simulink model "lego_selfbalance_custom"  (Simulink 8.2)
settings: Solver=ode3  SolverMode=SingleTasking  StartTime=0.0  StopTime=inf  FixedStep=0.004  MaxStep=TS  RelTol=1e-3
PostLoadFcn:
  | lego_selfbalance_plant;
  | lego_selfbalance_controller;
  | lego_selfbalance_simulation;
InitFcn:
  | lego_selfbalance_plant;
  | lego_selfbalance_controller;
  | lego_selfbalance_simulation;
  | 
  | lego_drive_selfbalance_InitData.mdl = get_param(bdroot,'Name');
  | lego_drive_selfbalance_InitData.cs = getActiveConfigSet(lego_drive_selfbalance_InitData.mdl);
values from neighbouring files (symbols this model uses):
  A1 = [ ... (first row only)    [lego_selfbalance_plant.m]
  A2 = [ ... (first row only)    [lego_selfbalance_plant.m]
  B1 = [ ... (first row only)    [lego_selfbalance_plant.m]
  B2 = [ ... (first row only)    [lego_selfbalance_plant.m]
  BATTERY = 8000    [lego_selfbalance_simulation.m]
  C1 = eye(4)    [lego_selfbalance_plant.m]
  C2 = eye(2)    [lego_selfbalance_plant.m]
  D = 0.04    [lego_selfbalance_plant.m]
  D1 = zeros(4, 2)    [lego_selfbalance_plant.m]
  D2 = zeros(2)    [lego_selfbalance_plant.m]
  GYRO0 = 600    [lego_selfbalance_simulation.m]
  R = 0.04    [lego_selfbalance_plant.m]
  START_POS = [100, 100]    [lego_selfbalance_simulation.m]
  TS = 0.001    [lego_selfbalance_simulation.m]
  W = 0.14    [lego_selfbalance_plant.m]
  X1IV = [ ... (first row only)    [lego_selfbalance_simulation.m]
  X2IV = [ ... (first row only)    [lego_selfbalance_simulation.m]
undefined symbols (not defined in the file or in its folder): a_b, a_d, a_gc, a_gd, a_r, DiscIntNeverNeededParam, k_f, k_i, k_sync, pwm_gain, pwm_offset, time_start, ts1, Turn
libraries: legonxtlib x11, simulink x4, realtime_examples_misc x1
PreSaveFcn:
  | set_param(gcs, 'Location',[35 56 895 605])
CloseFcn:
  | clear lego_drive_selfbalance_InitData
  | lego_selfbalance_closemodel
settings Model: Creator=The MathWorks Inc.  LastModifiedBy=Alphonso Monk  ExtModeTrigDuration=2
settings OptimizationCC: OptimizeModelRefInitCode=on  LifeSpan=1
settings DebuggingCC: SolverPrmCheckMsg=none  SingleTaskRateTransMsg=warning  Int32ToFloatConvMsg=none  ParameterPrecisionLossMsg=none
settings HardwareCC: ProdLargestAtomicInteger=Long  ProdLargestAtomicFloat=Float  ProdEndianess=LittleEndian  ProdHWDeviceType=ARM Compatible->ARM 7
settings SFSimCC: SimParseCustomCode=off
settings RTWCC: SystemTargetFile=realtime.tlc  GenCodeOnly=on  GenerateMakefile=off  TemplateMakefile=realtime.tmf  Description=Run on Target Hardware  RTWVerbose=off  ProcessScript=realtime_make_rtw_hook
settings CodeAppCC: CustomSymbolStrType=$N$R$M  InternalIdentifier=Classic
settings STFCustomTargetCC: TargetLibSuffix=.a  CodeReplacementLibrary=ANSI_C  GenerateSampleERTMain=on  ERTCustomFileBanners=on  SupportNonInlinedSFcns=off  SupportVariableSizeSignals=on  MATLABClassNameForMDSCustomization=Simulink.SoftwareTarget.ERTCustomization  GRTInterface=off  SystemTargetFile=realtime.tlc
settings ERTTargetCC: CodeReplacementLibrary=ANSI_C  MultiwordLength=2048  GenerateSampleERTMain=on  ParMdlRefBuildCompliant=off  CompOptLevelCompliant=off  ConcurrentExecutionCompliant=off  CombineOutputUpdateFcns=off  ERTFirstTimeCompliant=off  SupportContinuousTime=on  SupportVariableSizeSignals=on  ModelStepFunctionPrototypeControlCompliant=off  CPPClassGenCompliant=off  ExtModeTransport=1  ExtModeMexFile=ext_serial_win32_comm_no_acks_rtt_byteswap  ExtModeMexArgs=0 16 9600  InlinedParameterPlacement=NonHierarchical  ERTSrcFileBannerTemplate=realtime_code_template.cgt  ERTHdrFileBannerTemplate=realtime_code_template.cgt  ERTDataSrcFileTemplate=realtime_code_template.cgt  ERTDataHdrFileTemplate=realtime_code_template.cgt  ERTCustomFileTemplate=realtime_file_process.tlc  ConvertIfToSwitch=off  SuppressUnreachableDefaultCases=off
settings SettingsController: Description=Run on Hardware Dialog  TargetExtensionPlatform=LEGO MINDSTORMS NXT
settings MATStruct: Find_com_port=[0.0]  Enable_overrun_detection=[0.0]  Enable_LEGO_to_LEGO_communication=[1.0]  Bluetooth_mode=[1.0]  Slave_bluetooth_address=00:16:53:0f:0c:09

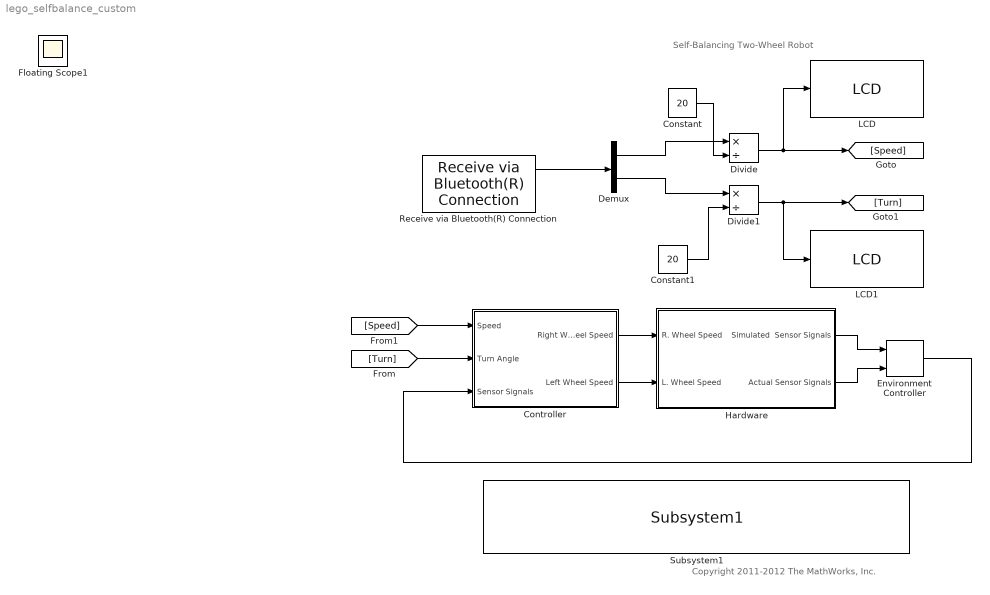
== system lego_selfbalance_custom ==
  note: Copyright 2011-2012 The MathWorks, Inc.
  note: Self-Balancing Two-Wheel Robot
  Constant : Constant  Value=20
  Constant1 : Constant  Value=20
  Controller : Subsystem  TreatAsAtomicUnit=on
  Demux : Demux  Outputs=2
  Divide : Product  Inputs=*/  OutDataTypeStr=single
  Divide1 : Product  Inputs=*/  OutDataTypeStr=single
  Environment Controller : simulink/Signal Routing/Environment Controller
  Hardware : Subsystem  VariantControl=DoSim
  LCD : legonxtlib/LCD  slcdStr=Speed  slcdLine=1  slcdFormat=Decimal
  LCD1 : legonxtlib/LCD  slcdStr=Turn:  slcdLine=2  slcdFormat=Decimal
  Receive via Bluetooth(R) Connection : legonxtlib/Receive via Bluetooth(R) Connection  mailbox=1  dataType=int32  dataSize=2  sampleTime=0.048
  Subsystem1 : realtime_examples_misc/Subsystem1  SystemSampleTime=-1
  Floating Scope1 : Scope
      settings: Floating=on  YMin=0  YMax=70000
  wires:
  Environment Controller/1 -> Controller/3(Sensor Signals)
  Controller/1(Right Wheel Speed) -> Hardware/1(R. Wheel Speed)
  Controller/2(Left Wheel Speed) -> Hardware/2(L. Wheel Speed)
  Hardware/1(Simulated  Sensor Signals) -> Environment Controller/1
  Hardware/2(Actual Sensor Signals) -> Environment Controller/2
  Constant/1 -> Divide/2
  Receive via Bluetooth(R) Connection/1 -> Demux/1
  Demux/1 -> Divide/1
  Constant1/1 -> Divide1/2
  Demux/2 -> Divide1/1
  Divide/1 -> [Speed], LCD/1
  Divide1/1 -> [Turn], LCD1/1
  [Turn] -> Controller/2(Turn Angle)
  [Speed] -> Controller/1(Speed)

== system lego_selfbalance_custom/Controller ==
  Speed : Inport
  Turn Angle : Inport  Port=2
  Sensor Signals : Inport  Port=3
  Balance and Drive Control : Subsystem
  Compare To Constant : simulink/Logic and Bit Operations/Compare To Constant  relop=>=  const=time_start  OutDataTypeStr=boolean
  Demux : Demux  Outputs=5
  Gyro Calibration : Subsystem  TreatAsAtomicUnit=on
  Logical Operator : Logic  Operator=NOT  AllPortsSameDT=off  OutDataTypeStr=boolean
  Right Wheel Speed : Outport
  Left Wheel Speed : Outport  Port=2
  wires:
  Compare To Constant/1 -> Logical Operator/1, Balance and Drive Control/Enable
  Gyro Calibration/1(Gyro Offset) -> Balance and Drive Control/1(Gyro Offset)
  Logical Operator/1 -> Gyro Calibration/Enable
  Sensor Signals/1 -> Demux/1
  Demux/4 -> Gyro Calibration/1(Gyro), Balance and Drive Control/2(Gyro)
  Speed/1 -> Balance and Drive Control/3(Speed)
  Turn Angle/1 -> Balance and Drive Control/4(Turn Angle)
  Demux/5 -> Balance and Drive Control/7(Battery)
  Demux/3 -> Balance and Drive Control/6(L. Wheel Rotation)
  Demux/2 -> Balance and Drive Control/5(R. Wheel Rotation)
  Demux/1 -> Compare To Constant/1
  Balance and Drive Control/1(R. Wheel Speed) -> Right Wheel Speed/1
  Balance and Drive Control/2(L. Wheel Speed) -> Left Wheel Speed/1

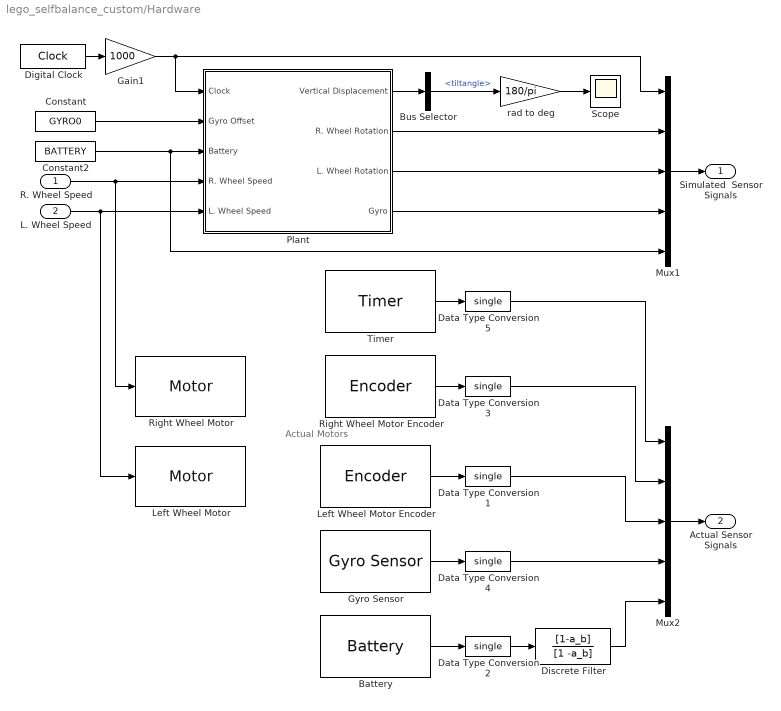
== system lego_selfbalance_custom/Hardware ==
  note: Actual
      | Motors
  R. Wheel Speed : Inport
  L. Wheel Speed : Inport  Port=2
  Battery : legonxtlib/Battery  sampleTime=ts1
  Bus Selector : BusSelector  OutputSignals=tiltangle
  Constant : Constant  Value=GYRO0  OutDataTypeStr=single
  Constant2 : Constant  Value=BATTERY  OutDataTypeStr=single
  Data Type Conversion{1..5} (5 alike) : DataTypeConversion  OutDataTypeStr=single  RndMeth=Simplest
  Digital Clock : DigitalClock  SampleTime=4*TS
  Discrete Filter : DiscreteFilter  Numerator=[1-a_b]  Denominator=[1 -a_b]
  Gain1 : Gain  Gain=1000  OutDataTypeStr=single  ParamDataTypeStr=Inherit: Same as input
  Gyro Sensor : legonxtlib/Gyro Sensor  portNumber=4  outputMode=Raw A/D (0 - 1023)  offset=600  sampleTime=ts1
  Left Wheel Motor : legonxtlib/Motor  sportNumber=C  sstopAction=Brake
  Left Wheel Motor Encoder : legonxtlib/Encoder  portNumber=C  opMode=No reset  sampleTime=ts1
  Mux1 : Mux  Inputs=5
  Mux2 : Mux  Inputs=5
  Plant : Subsystem
  Right Wheel Motor : legonxtlib/Motor  sportNumber=B  sstopAction=Brake
  Right Wheel Motor Encoder : legonxtlib/Encoder  portNumber=B  opMode=No reset  sampleTime=ts1
  Scope : Scope
      settings: YMin=-90  YMax=90
  Timer : legonxtlib/Timer  sampleTime=ts1
  rad to deg : Gain  Gain=180/pi
  Simulated  Sensor Signals : Outport
  Actual Sensor Signals : Outport  Port=2
  wires:
  Data Type Conversion5/1 -> Mux2/1
  Timer/1 -> Data Type Conversion5/1
  Data Type Conversion4/1 -> Mux2/4
  Data Type Conversion1/1 -> Mux2/3
  Data Type Conversion3/1 -> Mux2/2
  Mux2/1 -> Actual Sensor Signals/1
  Left Wheel Motor Encoder/1 -> Data Type Conversion1/1
  Right Wheel Motor Encoder/1 -> Data Type Conversion3/1
  Battery/1 -> Data Type Conversion2/1
  Data Type Conversion2/1 -> Discrete Filter/1
  Discrete Filter/1 -> Mux2/5
  Gyro Sensor/1 -> Data Type Conversion4/1
  L. Wheel Speed/1 -> Plant/5(L. Wheel Speed), Left Wheel Motor/1
  Mux1/1 -> Simulated  Sensor Signals/1
  Plant/3(L. Wheel Rotation) -> Mux1/3
  R. Wheel Speed/1 -> Plant/4(R. Wheel Speed), Right Wheel Motor/1
  Constant2/1 -> Mux1/5, Plant/3(Battery)
  Plant/2(R. Wheel Rotation) -> Mux1/2
  Plant/4(Gyro) -> Mux1/4
  Digital Clock/1 -> Gain1/1
  Gain1/1 -> Mux1/1, Plant/1(Clock)
  rad to deg/1 -> Scope/1
  Plant/1(Vertical Displacement) -> Bus Selector/1
  Bus Selector/1 -> rad to deg/1  "<tiltangle>"
  Constant/1 -> Plant/2(Gyro Offset)

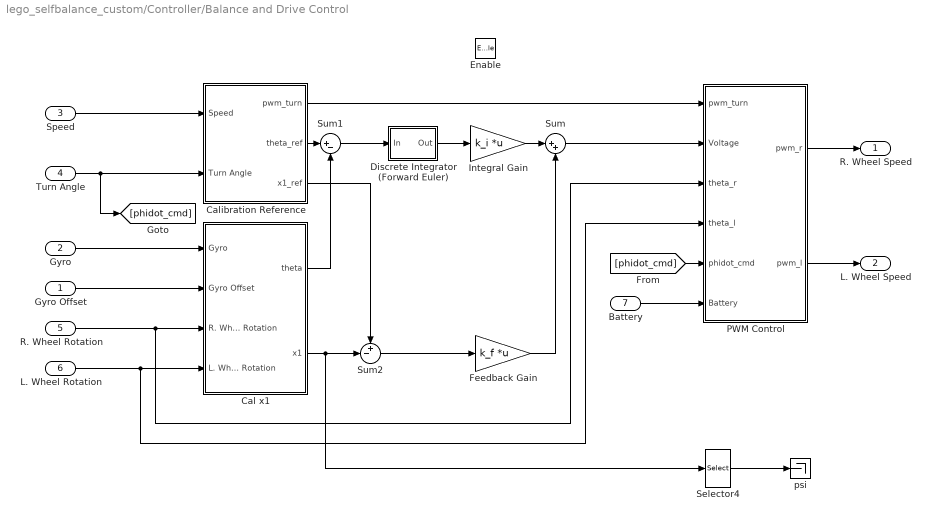
== system lego_selfbalance_custom/Controller/Balance and Drive Control ==
  Gyro Offset : Inport
  Gyro : Inport  Port=2
  Speed : Inport  Port=3
  Turn Angle : Inport  Port=4
  R. Wheel Rotation : Inport  Port=5
  L. Wheel Rotation : Inport  Port=6
  Battery : Inport  Port=7
  Enable : EnablePort
  Cal x1 : Subsystem
  Calibration Reference : Subsystem
  Discrete Integrator (Forward Euler) : Subsystem
  Feedback Gain : Gain  Gain=k_f  Multiplication=Matrix(K*u)  OutDataTypeStr=Inherit: Same as input  ParamDataTypeStr=Inherit: Same as input
  Integral Gain : Gain  Gain=k_i  Multiplication=Matrix(K*u)  OutDataTypeStr=Inherit: Same as input  ParamDataTypeStr=Inherit: Same as input
  PWM Control : Subsystem
  Selector4 : Selector  InputPortWidth=4  IndexOptions=Index vector (dialog)  Indices=2  OutputSizes=1
  Sum : Sum  Inputs=|++  OutDataTypeStr=Inherit: Same as first input
  Sum1 : Sum  Inputs=|+-  OutDataTypeStr=Inherit: Same as first input
  Sum2 : Sum  Inputs=+-|  OutDataTypeStr=Inherit: Same as first input
  psi : Terminator
  R. Wheel Speed : Outport
  L. Wheel Speed : Outport  Port=2
  wires:
  [phidot_cmd] -> PWM Control/5(phidot_cmd)
  Selector4/1 -> psi/1
  Calibration Reference/3(x1_ref) -> Sum2/1
  Sum2/1 -> Feedback Gain/1
  Cal x1/2(x1) -> Selector4/1, Sum2/2
  Integral Gain/1 -> Sum/1
  Discrete Integrator (Forward Euler)/1(Out) -> Integral Gain/1
  Sum1/1 -> Discrete Integrator (Forward Euler)/1(In)
  Cal x1/1(theta) -> Sum1/2
  Calibration Reference/2(theta_ref) -> Sum1/1
  Feedback Gain/1 -> Sum/2
  L. Wheel Rotation/1 -> PWM Control/4(theta_l), Cal x1/4(L. Wheel Rotation)
  Battery/1 -> PWM Control/6(Battery)
  Sum/1 -> PWM Control/2(Voltage)
  Turn Angle/1 -> [phidot_cmd], Calibration Reference/2(Turn Angle)
  Speed/1 -> Calibration Reference/1(Speed)
  Calibration Reference/1(pwm_turn) -> PWM Control/1(pwm_turn)
  PWM Control/1(pwm_r) -> R. Wheel Speed/1
  PWM Control/2(pwm_l) -> L. Wheel Speed/1
  R. Wheel Rotation/1 -> PWM Control/3(theta_r), Cal x1/3(R. Wheel Rotation)
  Gyro/1 -> Cal x1/1(Gyro)
  Gyro Offset/1 -> Cal x1/2(Gyro Offset)

== system lego_selfbalance_custom/Controller/Gyro Calibration ==
  note: Calculate gyro offset
  Gyro : Inport
  Enable : EnablePort
  Constant : Constant  Value=440  OutDataTypeStr=uint32  SampleTime=0.2
  Gain2 : Gain  Gain=1-a_gc  OutDataTypeStr=Inherit: Same as input  ParamDataTypeStr=Inherit: Same as input
  Gain3 : Gain  Gain=a_gc  OutDataTypeStr=Inherit: Same as input  ParamDataTypeStr=Inherit: Same as input
  Speaker : legonxtlib/Speaker  sinputMode=Frequency only  sspeakerFreq=100  sspeakerVolume=80  sspeakerDuration=100
  Sum1 : Sum  Inputs=|++  OutDataTypeStr=Inherit: Same as first input
  Unit Delay : UnitDelay  SampleTime=-1
  Gyro Offset : Outport
  wires:
  Gain3/1 -> Sum1/2
  Unit Delay/1 -> Gain3/1
  Sum1/1 -> Unit Delay/1, Gyro Offset/1
  Gain2/1 -> Sum1/1
  Gyro/1 -> Gain2/1
  Constant/1 -> Speaker/1

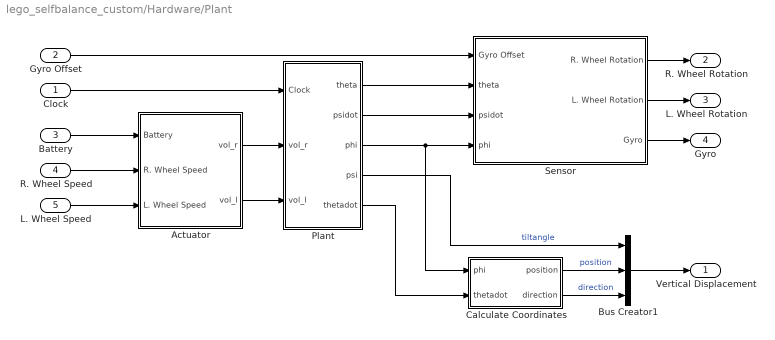
== system lego_selfbalance_custom/Hardware/Plant ==
  Clock : Inport
  Gyro Offset : Inport  Port=2
  Battery : Inport  Port=3
  R. Wheel Speed : Inport  Port=4
  L. Wheel Speed : Inport  Port=5
  Actuator : Subsystem
  Bus Creator1 : BusCreator  Inputs=3
  Calculate Coordinates : Subsystem
  Plant : Subsystem
  Sensor : Subsystem
  Vertical Displacement : Outport
  R. Wheel Rotation : Outport  Port=2
  L. Wheel Rotation : Outport  Port=3
  Gyro : Outport  Port=4
  wires:
  Clock/1 -> Plant/1(Clock)
  Plant/4(psi) -> Bus Creator1/1  "tiltangle"
  Bus Creator1/1 -> Vertical Displacement/1
  Calculate Coordinates/2(direction) -> Bus Creator1/3  "direction"
  Calculate Coordinates/1(position) -> Bus Creator1/2  "position"
  Plant/3(phi) -> Calculate Coordinates/1(phi), Sensor/4(phi)
  L. Wheel Speed/1 -> Actuator/3(L. Wheel Speed)
  Plant/5(thetadot) -> Calculate Coordinates/2(thetadot)
  Sensor/3(Gyro) -> Gyro/1
  R. Wheel Speed/1 -> Actuator/2(R. Wheel Speed)
  Sensor/2(L. Wheel Rotation) -> L. Wheel Rotation/1
  Sensor/1(R. Wheel Rotation) -> R. Wheel Rotation/1
  Gyro Offset/1 -> Sensor/1(Gyro Offset)
  Battery/1 -> Actuator/1(Battery)
  Plant/1(theta) -> Sensor/2(theta)
  Plant/2(psidot) -> Sensor/3(psidot)
  Actuator/2(vol_l) -> Plant/3(vol_l)
  Actuator/1(vol_r) -> Plant/2(vol_r)

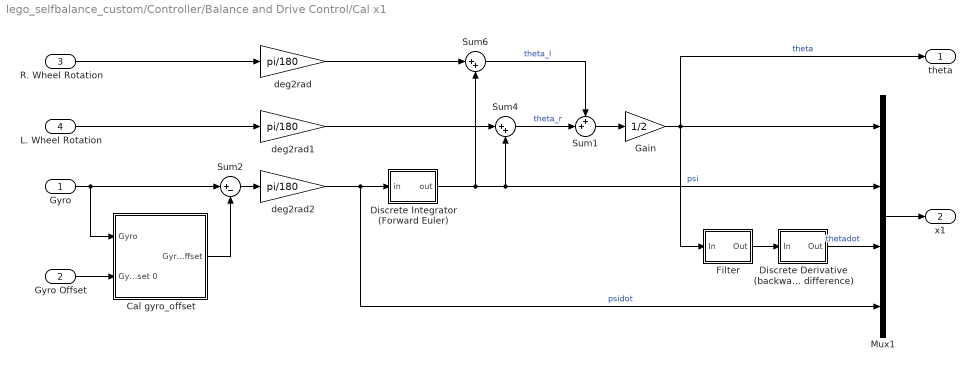
== system lego_selfbalance_custom/Controller/Balance and Drive Control/Cal x1 ==
  Gyro : Inport
  Gyro Offset : Inport  Port=2
  R. Wheel Rotation : Inport  Port=3
  L. Wheel Rotation : Inport  Port=4
  Cal gyro_offset : Subsystem
  Discrete Derivative (backward difference) : Subsystem
  Discrete Integrator (Forward Euler) : Subsystem
  Filter : Subsystem
  Gain : Gain  Gain=1/2  OutDataTypeStr=Inherit: Same as input  ParamDataTypeStr=Inherit: Same as input
  Mux1 : Mux
  Sum1 : Sum  Inputs=++|  OutDataTypeStr=Inherit: Same as first input
  Sum2 : Sum  Inputs=|+-  OutDataTypeStr=Inherit: Same as first input
  Sum4 : Sum  Inputs=|++  OutDataTypeStr=Inherit: Same as first input
  Sum6 : Sum  Inputs=|++  OutDataTypeStr=Inherit: Same as first input
  deg2rad : Gain  Gain=pi/180  OutDataTypeStr=Inherit: Same as input  ParamDataTypeStr=Inherit: Same as input
  deg2rad1 : Gain  Gain=pi/180  OutDataTypeStr=Inherit: Same as input  ParamDataTypeStr=Inherit: Same as input
  deg2rad2 : Gain  Gain=pi/180  OutDataTypeStr=Inherit: Same as input  ParamDataTypeStr=Inherit: Same as input
  theta : Outport
  x1 : Outport  Port=2
  wires:
  Gain/1 -> Mux1/1, theta/1, Filter/1(In)  "theta"
  Filter/1(Out) -> Discrete Derivative (backward difference)/1(In)
  deg2rad2/1 -> Mux1/4, Discrete Integrator (Forward Euler)/1(in)  "psidot"
  Sum1/1 -> Gain/1
  Sum4/1 -> Sum1/2  "theta_r"
  Sum6/1 -> Sum1/1  "theta_l"
  Discrete Derivative (backward difference)/1(Out) -> Mux1/3  "thetadot"
  L. Wheel Rotation/1 -> deg2rad1/1
  R. Wheel Rotation/1 -> deg2rad/1
  deg2rad/1 -> Sum6/1
  Discrete Integrator (Forward Euler)/1(out) -> Mux1/2, Sum4/2, Sum6/2  "psi"
  Mux1/1 -> x1/1
  deg2rad1/1 -> Sum4/1
  Gyro/1 -> Sum2/1, Cal gyro_offset/1(Gyro)
  Sum2/1 -> deg2rad2/1
  Cal gyro_offset/1(Gyro Offset) -> Sum2/2
  Gyro Offset/1 -> Cal gyro_offset/2(Gyro Offset 0)

== system lego_selfbalance_custom/Controller/Balance and Drive Control/Calibration Reference ==
  note: thetadot_cmd should be
      | between 0 and 7.5
  note: phidot_cmd should be
      | between 0 and 25
  Speed : Inport
  Turn Angle : Inport  Port=2
  Constant2 : Constant  Value=0  VectorParams1D=off  OutDataTypeStr=single
  Constant3 : Constant  Value=0  VectorParams1D=off  OutDataTypeStr=single
  Discrete Integrator (Forward Euler) : Subsystem
  Filter : Subsystem
  Mux : Mux
  pwm_turn : Outport
  theta_ref : Outport  Port=2
  x1_ref : Outport  Port=3
  wires:
  Filter/1(out) -> Mux/3, Discrete Integrator (Forward Euler)/1(in)  "thetadot_ref"
  Constant3/1 -> Mux/4  "psidot_ref"
  Constant2/1 -> Mux/2  "psi_ref"
  Discrete Integrator (Forward Euler)/1(out) -> Mux/1, theta_ref/1  "theta_ref"
  Mux/1 -> x1_ref/1
  Turn Angle/1 -> pwm_turn/1
  Speed/1 -> Filter/1(in)

== system lego_selfbalance_custom/Controller/Balance and Drive Control/Discrete Integrator (Forward Euler) ==
  In : Inport
  Gain : Gain  Gain=ts1  OutDataTypeStr=Inherit: Same as input  ParamDataTypeStr=Inherit: Same as input
  Sum : Sum  Inputs=|++  OutDataTypeStr=Inherit: Same as first input
  Unit Delay : UnitDelay  SampleTime=-1
  Out : Outport
  wires:
  In/1 -> Gain/1
  Sum/1 -> Unit Delay/1
  Gain/1 -> Sum/1
  Unit Delay/1 -> Out/1, Sum/2

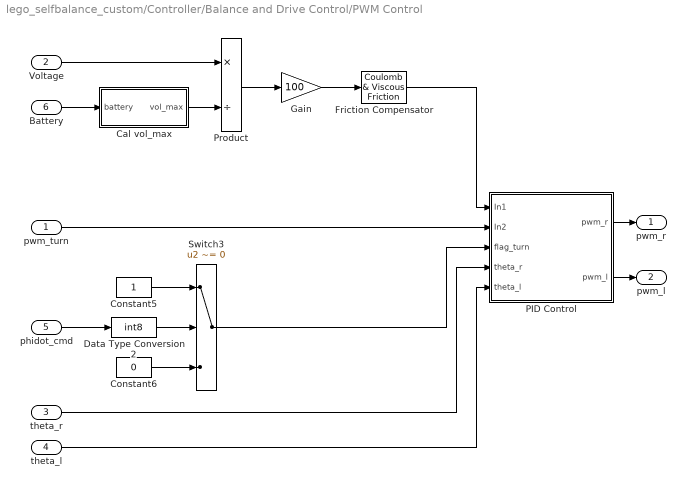
== system lego_selfbalance_custom/Controller/Balance and Drive Control/PWM Control ==
  pwm_turn : Inport
  Voltage : Inport  Port=2
  theta_r : Inport  Port=3
  theta_l : Inport  Port=4
  phidot_cmd : Inport  Port=5
  Battery : Inport  Port=6
  Cal vol_max : Subsystem
  Constant5 : Constant  OutDataTypeStr=boolean
  Constant6 : Constant  Value=0  OutDataTypeStr=boolean
  Data Type Conversion2 : DataTypeConversion  OutDataTypeStr=int8  RndMeth=Simplest
  Friction Compensator : simulink/Discontinuities/Coulomb & Viscous Friction  offset=pwm_offset  gain=pwm_gain
      settings: AttributesFormatString=gain = %<gain>\noffset = %<offset>
  Gain : Gain  Gain=100  OutDataTypeStr=Inherit: Same as input  ParamDataTypeStr=Inherit: Same as input
  PID Control : Subsystem
  Product : Product  Inputs=*/  RndMeth=Simplest  OutDataTypeStr=Inherit: Same as first input
  Switch3 : Switch  Criteria=u2 ~= 0
  pwm_r : Outport
  pwm_l : Outport  Port=2
  wires:
  Data Type Conversion2/1 -> Switch3/2
  phidot_cmd/1 -> Data Type Conversion2/1
  Constant6/1 -> Switch3/3
  Constant5/1 -> Switch3/1
  theta_l/1 -> PID Control/5(theta_l)
  theta_r/1 -> PID Control/4(theta_r)
  Cal vol_max/1(vol_max) -> Product/2
  Battery/1 -> Cal vol_max/1(battery)
  Product/1 -> Gain/1
  Voltage/1 -> Product/1
  Gain/1 -> Friction Compensator/1
  PID Control/1(pwm_r) -> pwm_r/1
  Friction Compensator/1 -> PID Control/1(In1)
  PID Control/2(pwm_l) -> pwm_l/1
  pwm_turn/1 -> PID Control/2(In2)
  Switch3/1 -> PID Control/3(flag_turn)

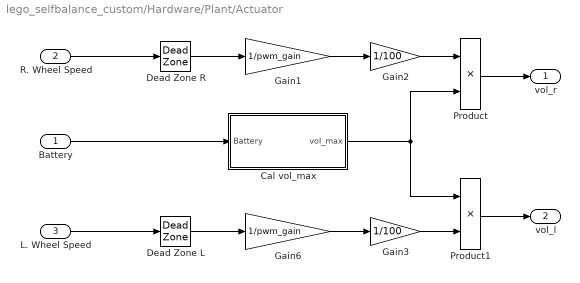
== system lego_selfbalance_custom/Hardware/Plant/Actuator ==
  Battery : Inport
  R. Wheel Speed : Inport  Port=2
  L. Wheel Speed : Inport  Port=3
  Cal vol_max : Subsystem
  Dead Zone L : DeadZone  LowerValue=-pwm_offset  UpperValue=pwm_offset  SaturateOnIntegerOverflow=on
      settings: AttributesFormatString=start=%<LowerValue>\nend=%<UpperValue>
  Dead Zone R : DeadZone  LowerValue=-pwm_offset  UpperValue=pwm_offset  SaturateOnIntegerOverflow=on
      settings: AttributesFormatString=start=%<LowerValue>\nend=%<UpperValue>
  Gain1 : Gain  Gain=1/pwm_gain  OutDataTypeStr=Inherit: Same as input  ParamDataTypeStr=Inherit: Same as input
  Gain2 : Gain  Gain=1/100  OutDataTypeStr=Inherit: Same as input  ParamDataTypeStr=Inherit: Same as input
  Gain3 : Gain  Gain=1/100  OutDataTypeStr=Inherit: Same as input  ParamDataTypeStr=Inherit: Same as input
  Gain6 : Gain  Gain=1/pwm_gain  OutDataTypeStr=Inherit: Same as input  ParamDataTypeStr=Inherit: Same as input
  Product : Product  RndMeth=Simplest
  Product1 : Product  RndMeth=Simplest
  vol_r : Outport
  vol_l : Outport  Port=2
  wires:
  Battery/1 -> Cal vol_max/1(Battery)
  Cal vol_max/1(vol_max) -> Product1/1, Product/2
  Dead Zone R/1 -> Gain1/1
  Product1/1 -> vol_l/1
  Gain3/1 -> Product1/2
  Product/1 -> vol_r/1
  Gain2/1 -> Product/1
  Gain6/1 -> Gain3/1
  Gain1/1 -> Gain2/1
  L. Wheel Speed/1 -> Dead Zone L/1
  R. Wheel Speed/1 -> Dead Zone R/1
  Dead Zone L/1 -> Gain6/1

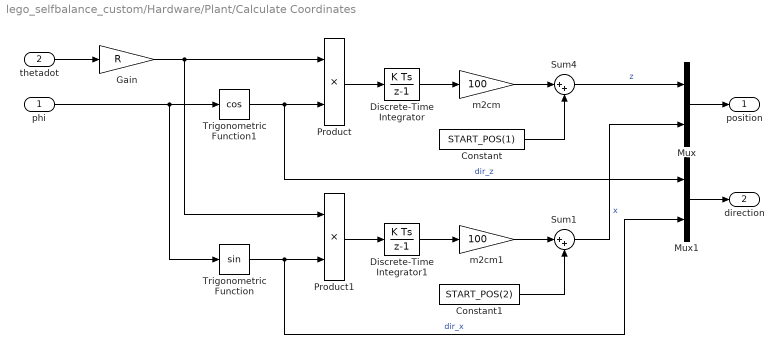
== system lego_selfbalance_custom/Hardware/Plant/Calculate Coordinates ==
  phi : Inport
  thetadot : Inport  Port=2
  Constant : Constant  Value=START_POS(1)  OutDataTypeStr=double
      settings: AttributesFormatString=DataType = %<OutDataTypeStr>
  Constant1 : Constant  Value=START_POS(2)  OutDataTypeStr=double
      settings: AttributesFormatString=DataType = %<OutDataTypeStr>
  Discrete-Time Integrator : DiscreteIntegrator  SampleTime=4*TS  ICPrevOutput=DiscIntNeverNeededParam  ICPrevScaledInput=DiscIntNeverNeededParam
  Discrete-Time Integrator1 : DiscreteIntegrator  SampleTime=4*TS  ICPrevOutput=DiscIntNeverNeededParam  ICPrevScaledInput=DiscIntNeverNeededParam
  Gain : Gain  Gain=R
  Mux : Mux  Inputs=2
  Mux1 : Mux  Inputs=2
  Product : Product  OutDataTypeStr=double  RndMeth=Simplest
  Product1 : Product  OutDataTypeStr=double  RndMeth=Simplest
  Sum1 : Sum  Inputs=|++
  Sum4 : Sum  Inputs=|++
  Trigonometric Function : Trigonometry
  Trigonometric Function1 : Trigonometry  Operator=cos
  m2cm : Gain  Gain=100
  m2cm1 : Gain  Gain=100
  position : Outport
  direction : Outport  Port=2
  wires:
  Mux1/1 -> direction/1
  Mux/1 -> position/1
  Sum1/1 -> Mux/2  "x"
  Constant1/1 -> Sum1/2
  m2cm1/1 -> Sum1/1
  Constant/1 -> Sum4/2
  Sum4/1 -> Mux/1  "z"
  m2cm/1 -> Sum4/1
  Gain/1 -> Product/1, Product1/1
  Discrete-Time Integrator1/1 -> m2cm1/1
  Discrete-Time Integrator/1 -> m2cm/1
  phi/1 -> Trigonometric Function/1, Trigonometric Function1/1
  thetadot/1 -> Gain/1
  Trigonometric Function1/1 -> Mux1/1, Product/2  "dir_z"
  Product/1 -> Discrete-Time Integrator/1
  Trigonometric Function/1 -> Mux1/2, Product1/2  "dir_x"
  Product1/1 -> Discrete-Time Integrator1/1

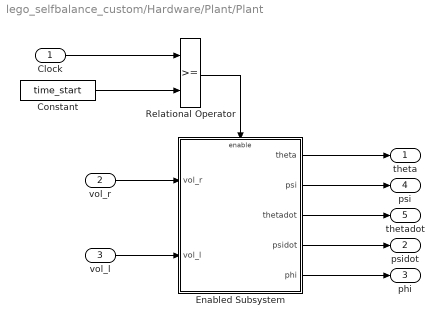
== system lego_selfbalance_custom/Hardware/Plant/Plant ==
  Clock : Inport
  vol_r : Inport  Port=2
  vol_l : Inport  Port=3
  Constant : Constant  Value=time_start  OutDataTypeStr=single
  Enabled Subsystem : Subsystem  TreatAsAtomicUnit=on
      settings: MinAlgLoopOccurrences=on
  Relational Operator : RelationalOperator  OutDataTypeStr=boolean
  theta : Outport
  psidot : Outport  Port=2
  phi : Outport  Port=3
  psi : Outport  Port=4
  thetadot : Outport  Port=5
  wires:
  Enabled Subsystem/4(psidot) -> psidot/1
  Enabled Subsystem/5(phi) -> phi/1
  Enabled Subsystem/2(psi) -> psi/1
  Enabled Subsystem/3(thetadot) -> thetadot/1
  Enabled Subsystem/1(theta) -> theta/1
  Constant/1 -> Relational Operator/2
  Clock/1 -> Relational Operator/1
  Relational Operator/1 -> Enabled Subsystem/Enable
  vol_l/1 -> Enabled Subsystem/2(vol_l)
  vol_r/1 -> Enabled Subsystem/1(vol_r)

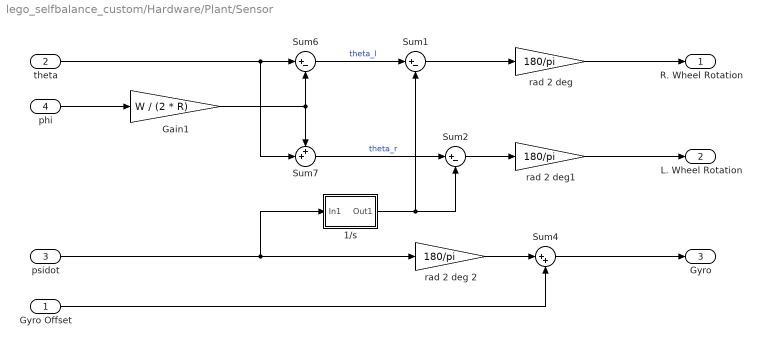
== system lego_selfbalance_custom/Hardware/Plant/Sensor ==
  Gyro Offset : Inport
  theta : Inport  Port=2
  psidot : Inport  Port=3
  phi : Inport  Port=4
  1/s : Subsystem
  Gain1 : Gain  Gain=W / (2 * R)
  Sum1 : Sum  Inputs=|+-
  Sum2 : Sum  Inputs=|+-
  Sum4 : Sum  Inputs=|++
  Sum6 : Sum  Inputs=|+-
  Sum7 : Sum  Inputs=++|
  rad 2 deg : Gain  Gain=180/pi  OutDataTypeStr=single
  rad 2 deg 2 : Gain  Gain=180/pi
  rad 2 deg1 : Gain  Gain=180/pi  OutDataTypeStr=single
  R. Wheel Rotation : Outport
  L. Wheel Rotation : Outport  Port=2
  Gyro : Outport  Port=3
  wires:
  1/s/1(Out1) -> Sum1/2, Sum2/2
  Sum6/1 -> Sum1/1  "theta_l"
  rad 2 deg1/1 -> L. Wheel Rotation/1
  rad 2 deg/1 -> R. Wheel Rotation/1
  Sum2/1 -> rad 2 deg1/1
  psidot/1 -> 1/s/1(In1), rad 2 deg 2/1
  Sum1/1 -> rad 2 deg/1
  Gain1/1 -> Sum6/2, Sum7/1
  phi/1 -> Gain1/1
  theta/1 -> Sum6/1, Sum7/2
  rad 2 deg 2/1 -> Sum4/1
  Sum7/1 -> Sum2/1  "theta_r"
  Gyro Offset/1 -> Sum4/2
  Sum4/1 -> Gyro/1

== system lego_selfbalance_custom/Controller/Balance and Drive Control/Cal x1/Cal gyro_offset ==
  Gyro : Inport
  Gyro Offset 0 : Inport  Port=2
  Gain1 : Gain  Gain=1-a_gd  OutDataTypeStr=Inherit: Same as input  ParamDataTypeStr=Inherit: Same as input
  Gain4 : Gain  Gain=a_gd  OutDataTypeStr=Inherit: Same as input  ParamDataTypeStr=Inherit: Same as input
  Sum2 : Sum  Inputs=|++  OutDataTypeStr=Inherit: Same as first input
  Unit Delay External IC : simulink/Additional Math & Discrete/Additional Discrete/Unit Delay External IC  tsamp=-1
  Gyro Offset : Outport
  wires:
  Gyro/1 -> Gain1/1
  Gyro Offset 0/1 -> Unit Delay External IC/2
  Gain1/1 -> Sum2/1
  Sum2/1 -> Gyro Offset/1, Unit Delay External IC/1
  Unit Delay External IC/1 -> Gain4/1
  Gain4/1 -> Sum2/2

== system lego_selfbalance_custom/Controller/Balance and Drive Control/Cal x1/Discrete Derivative (backward difference) ==
  In : Inport
  Gain : Gain  Gain=1/ts1  OutDataTypeStr=Inherit: Same as input  ParamDataTypeStr=Inherit: Same as input
  Sum : Sum  Inputs=|+-  OutDataTypeStr=Inherit: Same as first input
  Unit Delay : UnitDelay  SampleTime=-1
  Out : Outport
  wires:
  Gain/1 -> Out/1
  In/1 -> Sum/1, Unit Delay/1
  Unit Delay/1 -> Sum/2
  Sum/1 -> Gain/1

== system lego_selfbalance_custom/Controller/Balance and Drive Control/Cal x1/Discrete Integrator (Forward Euler) ==
  in : Inport
  Gain : Gain  Gain=ts1  OutDataTypeStr=Inherit: Same as input  ParamDataTypeStr=Inherit: Same as input
  Sum : Sum  Inputs=|++  OutDataTypeStr=Inherit: Same as first input
  Unit Delay : UnitDelay  SampleTime=-1
  out : Outport
  wires:
  Unit Delay/1 -> Sum/2, out/1
  Gain/1 -> Sum/1
  Sum/1 -> Unit Delay/1
  in/1 -> Gain/1

== system lego_selfbalance_custom/Controller/Balance and Drive Control/Cal x1/Filter ==
  In : Inport
  Gain2 : Gain  Gain=a_d  OutDataTypeStr=Inherit: Same as input  ParamDataTypeStr=Inherit: Same as input
  Gain3 : Gain  Gain=1-a_d  OutDataTypeStr=Inherit: Same as input  ParamDataTypeStr=Inherit: Same as input
  Sum : Sum  Inputs=|++  OutDataTypeStr=Inherit: Same as first input
  Unit Delay : UnitDelay  SampleTime=-1
  Out : Outport
  wires:
  In/1 -> Gain3/1
  Gain3/1 -> Sum/1
  Gain2/1 -> Sum/2
  Unit Delay/1 -> Gain2/1
  Sum/1 -> Out/1, Unit Delay/1

== system lego_selfbalance_custom/Controller/Balance and Drive Control/Calibration Reference/Discrete Integrator (Forward Euler) ==
  in : Inport
  Gain : Gain  Gain=ts1  OutDataTypeStr=Inherit: Same as input  ParamDataTypeStr=Inherit: Same as input
  Sum : Sum  Inputs=|++  OutDataTypeStr=Inherit: Same as first input
  Unit Delay : UnitDelay  SampleTime=-1
  out : Outport
  wires:
  in/1 -> Gain/1
  Sum/1 -> Unit Delay/1
  Gain/1 -> Sum/1
  Unit Delay/1 -> out/1, Sum/2

== system lego_selfbalance_custom/Controller/Balance and Drive Control/Calibration Reference/Filter ==
  note: Filter Function:
      |               1-a_r
      |          ----------------
      |          1-a_r*z^(-1)
  in : Inport
  Gain2 : Gain  Gain=a_r  OutDataTypeStr=Inherit: Same as input  ParamDataTypeStr=Inherit: Same as input
  Gain3 : Gain  Gain=1-a_r  OutDataTypeStr=Inherit: Same as input  ParamDataTypeStr=Inherit: Same as input
  Sum : Sum  Inputs=|++  OutDataTypeStr=Inherit: Same as first input
  Unit Delay : UnitDelay  SampleTime=-1
  out : Outport
  wires:
  in/1 -> Gain3/1
  Gain3/1 -> Sum/1
  Gain2/1 -> Sum/2
  Unit Delay/1 -> Gain2/1
  Sum/1 -> out/1, Unit Delay/1

== system lego_selfbalance_custom/Controller/Balance and Drive Control/PWM Control/Cal vol_max ==
  battery : Inport
  Constant : Constant  Value=0.625  OutDataTypeStr=single
      settings: AttributesFormatString=DataType = %<OutDataTypeStr>
  Gain3 : Gain  Gain=0.001089  OutDataTypeStr=Inherit: Same as input  ParamDataTypeStr=Inherit: Same as input
  Sum2 : Sum  Inputs=|+-  OutDataTypeStr=Inherit: Same as first input
  vol_max : Outport
  wires:
  Gain3/1 -> Sum2/1
  Sum2/1 -> vol_max/1
  Constant/1 -> Sum2/2
  battery/1 -> Gain3/1

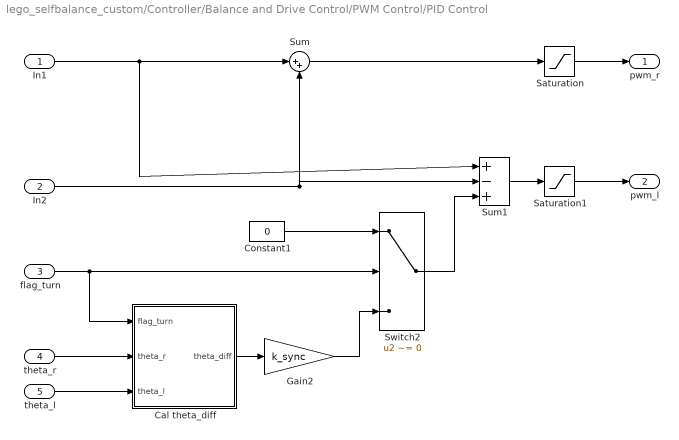
== system lego_selfbalance_custom/Controller/Balance and Drive Control/PWM Control/PID Control ==
  In1 : Inport
  In2 : Inport  Port=2
  flag_turn : Inport  Port=3
  theta_r : Inport  Port=4
  theta_l : Inport  Port=5
  Cal theta_diff : Subsystem
  Constant1 : Constant  Value=0  OutDataTypeStr=single
      settings: AttributesFormatString=DataType = %<OutDataTypeStr>
  Gain2 : Gain  Gain=k_sync  OutDataTypeStr=Inherit: Same as input  ParamDataTypeStr=Inherit: Same as input
  Saturation : Saturate  UpperLimit=100  LowerLimit=-100
      settings: AttributesFormatString=max = %<UpperLimit>\nmin = %<LowerLimit>
  Saturation1 : Saturate  UpperLimit=100  LowerLimit=-100
      settings: AttributesFormatString=max = %<UpperLimit>\nmin = %<LowerLimit>
  Sum : Sum  Inputs=|++  OutDataTypeStr=Inherit: Same as first input
  Sum1 : Sum  Inputs=|+-+  OutDataTypeStr=Inherit: Same as first input
  Switch2 : Switch  Criteria=u2 ~= 0
  pwm_r : Outport
  pwm_l : Outport  Port=2
  wires:
  In1/1 -> Sum1/1, Sum/1
  Gain2/1 -> Switch2/3
  Constant1/1 -> Switch2/1
  flag_turn/1 -> Switch2/2, Cal theta_diff/1(flag_turn)
  Cal theta_diff/1(theta_diff) -> Gain2/1
  Saturation/1 -> pwm_r/1
  Saturation1/1 -> pwm_l/1
  In2/1 -> Sum1/2, Sum/2
  Sum/1 -> Saturation/1
  theta_r/1 -> Cal theta_diff/2(theta_r)
  theta_l/1 -> Cal theta_diff/3(theta_l)
  Switch2/1 -> Sum1/3
  Sum1/1 -> Saturation1/1

== system lego_selfbalance_custom/Hardware/Plant/Actuator/Cal vol_max ==
  note: Calculate maximum DC motor (battery)
      | voltage using an experimental expression
  Battery : Inport
  Constant : Constant  Value=0.625  OutDataTypeStr=single
  Gain3 : Gain  Gain=0.001089  OutDataTypeStr=Inherit: Same as input  ParamDataTypeStr=Inherit: Same as input
  Sum2 : Sum  Inputs=|+-  OutDataTypeStr=Inherit: Same as first input
  vol_max : Outport
  wires:
  Constant/1 -> Sum2/2
  Sum2/1 -> vol_max/1
  Gain3/1 -> Sum2/1
  Battery/1 -> Gain3/1

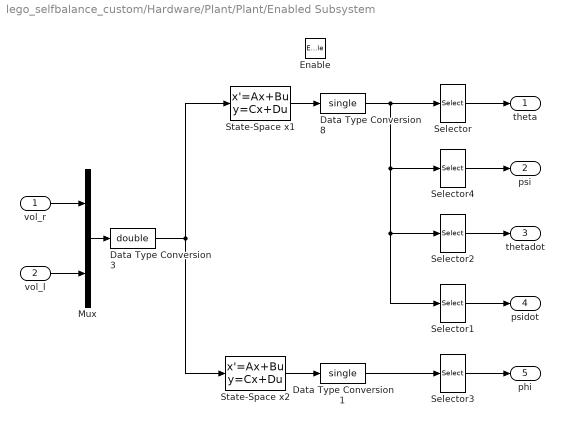
== system lego_selfbalance_custom/Hardware/Plant/Plant/Enabled Subsystem ==
  vol_r : Inport
  vol_l : Inport  Port=2
  Enable : EnablePort
  Data Type Conversion1 : DataTypeConversion  OutDataTypeStr=single  RndMeth=Nearest
  Data Type Conversion3 : DataTypeConversion  OutDataTypeStr=double  RndMeth=Nearest
  Data Type Conversion8 : DataTypeConversion  OutDataTypeStr=single  RndMeth=Nearest
  Mux : Mux  Inputs=2
  Selector : Selector  InputPortWidth=4  IndexOptions=Index vector (dialog)  Indices=1  OutputSizes=1
  Selector1 : Selector  InputPortWidth=4  IndexOptions=Index vector (dialog)  Indices=4  OutputSizes=1
  Selector2 : Selector  InputPortWidth=4  IndexOptions=Index vector (dialog)  Indices=3  OutputSizes=1
  Selector3 : Selector  InputPortWidth=2  IndexOptions=Index vector (dialog)  Indices=1  OutputSizes=1
  Selector4 : Selector  InputPortWidth=4  IndexOptions=Index vector (dialog)  Indices=2  OutputSizes=1
  State-Space x1 : StateSpace  A=A1  B=B1  C=C1  D=D1  X0=X1IV
  State-Space x2 : StateSpace  A=A2  B=B2  C=C2  D=D2  X0=X2IV
  theta : Outport  InitialOutput=0
  psi : Outport  Port=2  InitialOutput=0
  thetadot : Outport  Port=3  InitialOutput=0
  psidot : Outport  Port=4  InitialOutput=0
  phi : Outport  Port=5  InitialOutput=0
  wires:
  Data Type Conversion1/1 -> Selector3/1
  Data Type Conversion3/1 -> State-Space x1/1, State-Space x2/1
  Data Type Conversion8/1 -> Selector2/1, Selector1/1, Selector4/1, Selector/1
  Selector1/1 -> psidot/1
  Selector/1 -> theta/1
  Selector4/1 -> psi/1
  Selector2/1 -> thetadot/1
  Selector3/1 -> phi/1
  Mux/1 -> Data Type Conversion3/1
  vol_l/1 -> Mux/2
  vol_r/1 -> Mux/1
  State-Space x1/1 -> Data Type Conversion8/1
  State-Space x2/1 -> Data Type Conversion1/1

== system lego_selfbalance_custom/Hardware/Plant/Sensor/1/s ==
  In1 : Inport
  Data Type Conversion1 : DataTypeConversion  OutDataTypeStr=double  RndMeth=Nearest
      settings: AttributesFormatString=Round = %<RndMeth>
  Discrete-Time Integrator : DiscreteIntegrator  gainval=1  SampleTime=4*TS  ICPrevOutput=DiscIntNeverNeededParam  ICPrevScaledInput=DiscIntNeverNeededParam
  Out1 : Outport
  wires:
  In1/1 -> Data Type Conversion1/1
  Data Type Conversion1/1 -> Discrete-Time Integrator/1
  Discrete-Time Integrator/1 -> Out1/1

== system lego_selfbalance_custom/Controller/Balance and Drive Control/PWM Control/PID Control/Cal theta_diff ==
  note: Save the difference between
      | left and right motor revolution angle
  note: Detect turn -> straight run change
  note: When phidot goes to 0, remember the difference
      | between L and R encoder values (they need not be equal,
      | since robot would have been turning). While phidot == 0,
      | apply correction to maintain that difference.
      | If phidot ~= 0, don't apply the correction.
  flag_turn : Inport
  theta_r : Inport  Port=2
  theta_l : Inport  Port=3
  Detect Flag Falling : Subsystem
  Set theta_offset : Subsystem
  Sum1 : Sum  Inputs=|+-  OutDataTypeStr=Inherit: Same as first input
  Sum5 : Sum  Inputs=|-+  OutDataTypeStr=Inherit: Same as first input
  theta_diff : Outport
  wires:
  Set theta_offset/1(theta_offset) -> Sum5/1
  theta_l/1 -> Sum1/2
  theta_r/1 -> Sum1/1
  Sum1/1 -> Sum5/2, Set theta_offset/1(theta_diff)
  Detect Flag Falling/1(falling) -> Set theta_offset/Enable
  Sum5/1 -> theta_diff/1
  flag_turn/1 -> Detect Flag Falling/1(flag)

== system lego_selfbalance_custom/Controller/Balance and Drive Control/PWM Control/PID Control/Cal theta_diff/Detect Flag Falling ==
  flag : Inport
  Constant : Constant  Value=0  VectorParams1D=off  OutDataTypeStr=boolean
      settings: AttributesFormatString=DataType = %<OutDataTypeStr>
  Constant1 : Constant  VectorParams1D=off  OutDataTypeStr=boolean
      settings: AttributesFormatString=DataType = %<OutDataTypeStr>
  Logical Operator : Logic  AllPortsSameDT=off  OutDataTypeStr=boolean
  Relational Operator : RelationalOperator  Operator===  OutDataTypeStr=boolean
  Relational Operator1 : RelationalOperator  Operator===  OutDataTypeStr=boolean
  Unit Delay : UnitDelay  SampleTime=-1
  falling : Outport
  wires:
  Logical Operator/1 -> falling/1
  Relational Operator1/1 -> Logical Operator/2
  Relational Operator/1 -> Logical Operator/1
  Constant1/1 -> Relational Operator1/2
  Unit Delay/1 -> Relational Operator1/1
  Constant/1 -> Relational Operator/2
  flag/1 -> Relational Operator/1, Unit Delay/1

== system lego_selfbalance_custom/Controller/Balance and Drive Control/PWM Control/PID Control/Cal theta_diff/Set theta_offset ==
  theta_diff : Inport
  Enable : EnablePort
  theta_offset : Outport
  wires:
  theta_diff/1 -> theta_offset/1
